simulink model "demo_simiplified_2"  (R2022b)
settings: Solver=VariableStepAuto  StartTime=0.0  StopTime=sim_time  RelTol=1e-4  AbsTol=1e-4
model workspace (MATLAB code in the model file):
  | official_parameters_2
undefined symbols (not defined in the file or in its folder): cd1, cd2_1, cd2_2, gas_pipe_D, initial_system_T, mass_flow_cp, Max_tank_V, N2_T, sim_time, stack_area, stack_mea_rho, stack_num_cells, stack_num_channels, stack_t_gdl_A, stack_t_gdl_C, stack_t_membrane, stack_w_channels, tank_plant_area, water_pipe_D
libraries: fl_lib x25, nesl_utility x4, SimscapeFluids_lib x1
CloseFcn:
  | try,close(h1_ssc_electrolyzer),end
  | clear h1_ssc_electrolyzer
  | try,close(h2_ssc_electrolyzer),end
  | clear h2_ssc_electrolyzer
  | try,close(h3_ssc_electrolyzer),end
  | clear h3_ssc_electrolyzer
  | 
  | clear tout simlog_ssc_electrolyzer
Description:
  | PEM Electrolysis System
settings Model: Creator=The MathWorks, Inc.  LastModifiedBy=15713
settings SolverCC: AutoScaleAbsTol=off  MaxConsecutiveMinStep=8  AlgebraicLoopSolver=TrustRegion  MaxZcPerStep=1
settings DataIOCC: ReturnWorkspaceOutputs=off
settings DebuggingCC: UnconnectedInputMsg=warning  UnconnectedOutputMsg=warning  UnconnectedLineMsg=warning  SymbolicDimsDataTypeCodeGenerationDiagnostic=none  SFMachineParentedDataDiag=warning
settings ModelReferenceCC: EnableRefExpFcnMdlSchedulingChecks=on
settings SFSimCC: CustomCodeUndefinedFunction=UseInterfaceOnly
settings RTWCC: DLArmComputeVersion=19.05
settings SimscapeCC: SimscapeLogType=all  SimscapeLogSimulationStatistics=on  SimscapeLogName=simlog_ssc_electrolyzer  SimscapeLogDataHistory=10000

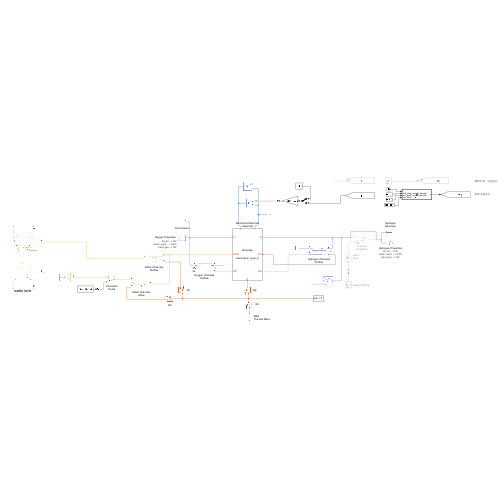
[thumbnail: Simulink's stored preview of the top-level diagram]
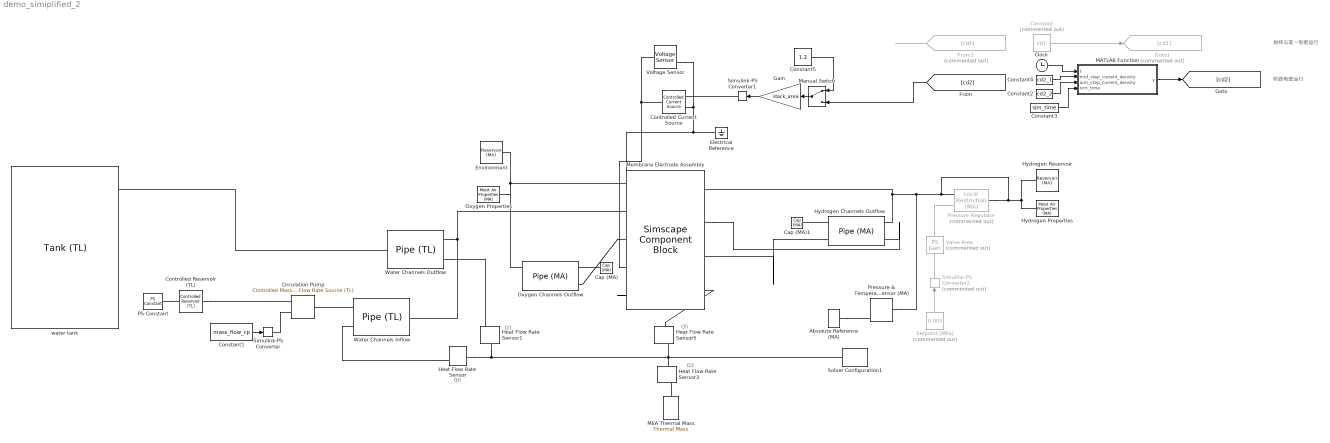
== system demo_simiplified_2 ==
  note: 始终以某一电密运行
  note: Q1
  note: Q0
  note: Q3
  note: Q5
  note: 阶跃电密运行
  Absolute Reference (MA) : fl_lib/Moist Air/Elements/Absolute Reference (MA)
  Cap (MA) : fl_lib/Moist Air/Elements/Cap (MA)  p_specify=off  p_priority=None  p=0.1 MPa  p_nominal_specify=off  p_nominal_unit=MPa  p_nominal_value=1  T_specify=off  T_priority=None  T=300 K  T_nominal_specify=off  T_nominal_unit=K  T_nominal_value=1  x_w_specify=off  x_w_priority=None  x_w=0  x_w_nominal_specify=off  x_w_nominal_unit=1  x_w_nominal_value=1  x_g_specify=off  x_g_priority=None  x_g=0  x_g_nominal_specify=off  x_g_nominal_unit=1  x_g_nominal_value=1
      settings: InternalSimscapePortConfiguration="{\"Bottom\":[],\"Left\":[{\"id\":\"A\",\"label\":\"\",\"type\":\"foundation.moist_air.moist_air\"}],\"Right\":[],\"Top\":[]}"
  Cap (MA)1 : fl_lib/Moist Air/Elements/Cap (MA)  p_specify=off  p_priority=None  p=0.1 MPa  p_nominal_specify=off  p_nominal_unit=MPa  p_nominal_value=1  T_specify=on  T_priority=High  T=initial_system_T degC  T_nominal_specify=off  T_nominal_unit=K  T_nominal_value=1  x_w_specify=off  x_w_priority=None  x_w=0  x_w_nominal_specify=off  x_w_nominal_unit=1  x_w_nominal_value=1  x_g_specify=off  x_g_priority=None  x_g=0  x_g_nominal_specify=off  x_g_nominal_unit=1  x_g_nominal_value=1
      settings: InternalSimscapePortConfiguration="{\"Bottom\":[],\"Left\":[{\"id\":\"A\",\"label\":\"\",\"type\":\"foundation.moist_air.moist_air\"}],\"Right\":[],\"Top\":[]}"
  Circulation Pump : fl_lib/Thermal Liquid/Sources/Controlled Mass Flow Rate Source (TL)  area=pi*water_pipe_D^2/4 m^2
      settings: InternalSimscapePortConfiguration="{\"Bottom\":[],\"Left\":[{\"id\":\"A\",\"label\":\"A\",\"type\":\"foundation.thermal_liquid.thermal_liquid\"},{\"id\":\"M\",\"label\":\"M\",\"type\":\"input\"}],\"Right\":[{\"id\":\"B\",\"label\":\"B\",\"type\":\"foundation.thermal_liquid.thermal_liquid\"}],\"Top\":[]}"
  Clock : Clock
  Constant : Constant  Commented=on  Value=cd1
  Constant1 : Constant  Value=mass_flow_cp
  Constant2 : Constant  Value=cd2_2
  Constant3 : Constant  Value=sim_time
  Constant4 : Constant  Value=cd2_1
  Constant5 : Constant  Value=1.2
  Controlled Current Source : fl_lib/Electrical/Electrical Sources/Controlled Current Source
  Controlled Reservoir (TL) : fl_lib/Thermal Liquid/Elements/Controlled Reservoir (TL)  pressure_spec=foundation.enum.pressure_spec.atmospheric  reservoir_pressure=0.101325 MPa  area=pi*water_pipe_D^2/4 m^2
      settings: InternalSimscapePortConfiguration="{\"Bottom\":[],\"Left\":[{\"id\":\"A\",\"label\":\"A\",\"type\":\"foundation.thermal_liquid.thermal_liquid\"}],\"Right\":[{\"id\":\"T_in\",\"label\":\"T\",\"type\":\"input\"}],\"Top\":[]}"
  Electrical Reference : fl_lib/Electrical/Electrical Elements/Electrical Reference
  Environment : fl_lib/Moist Air/Elements/Reservoir (MA)  pressure_spec=foundation.enum.pressure_spec.specified  reservoir_pressure=env_p MPa  temperature_spec=foundation.enum.temperature_spec.specified  reservoir_temperature=initial_system_T degC  moisture_spec=foundation.enum.moisture_spec.mole_fraction  reservoir_RH=0.5  reservoir_x_w=0.01  reservoir_y_w=0  reservoir_HR=0.01  trace_gas_spec=foundation.enum.trace_gas_spec.mole_fraction  reservoir_x_g=0.001  reservoir_y_g=1  RH_ws=1  area_A=pi*gas_pipe_D^2/4 m^2
  From1 : From  Commented=on  GotoTag=cd1
  Gain : Gain  Gain=stack_area
  Goto1 : Goto  Commented=on  GotoTag=cd1
  Heat Flow Rate Sensor{,1,3,5} (4 alike) : fl_lib/Thermal/Thermal Sensors/Heat Flow Rate Sensor
  Hydrogen Reservoir : fl_lib/Moist Air/Elements/Reservoir (MA)  pressure_spec=foundation.enum.pressure_spec.specified  reservoir_pressure=env_p MPa  temperature_spec=foundation.enum.temperature_spec.specified  reservoir_temperature=20 degC  moisture_spec=foundation.enum.moisture_spec.mole_fraction  reservoir_RH=0.5  reservoir_x_w=0.01  reservoir_y_w=0  reservoir_HR=0.01  trace_gas_spec=foundation.enum.trace_gas_spec.mole_fraction  reservoir_x_g=0.001  reservoir_y_g=1  RH_ws=1  area_A=pi*gas_pipe_D^2/4 m^2
  Hydrogen Channels Outflow : fl_lib/Moist Air/Elements/Pipe (MA)  length=sqrt(stack_area) cm  area=stack_w_channels^2 * stack_num_channels * stack_num_cells cm^2  Dh=stack_w_channels cm  length_add=1 cm  roughness=15e-6 m  Re_lam=2000  Re_tur=4000  shape_factor=64  Nu_lam=3.66  wall_condensation=simscape.enum.onoff.off  RH_ws=1  time_constant=1e-3 s  moisture_trace_gas_source=foundation.enum.moisture_trace_gas_source.controlled  moisture_source_spec=foundation.enum.moisture_source_spec.vapor  moisture_mass_flow=0 kg/s  moisture_temperature_spec=foundation.enum.temperature_spec.atmospheric  moisture_temperature=293.15 K  trace_gas_mass_flow=0 kg/s  trace_gas_temperature_spec=foundation.enum.temperature_spec.atmospheric  trace_gas_temperature=293.15 K  p_I_specify=on  p_I_priority=High  p_I=env_p MPa  p_I_nominal_specify=off  p_I_nominal_unit=MPa  p_I_nominal_value=1  T_I_specify=on  T_I_priority=High  T_I=initial_system_T degC  T_I_nominal_specify=off  T_I_nominal_unit=K  T_I_nominal_value=1  RH_I_specify=on  RH_I_priority=None  RH_I=0  RH_I_nominal_specify=off  RH_I_nominal_unit=1  RH_I_nominal_value=1  x_w_I_specify=off  x_w_I_priority=None  x_w_I=0  x_w_I_nominal_specify=off  x_w_I_nominal_unit=1  x_w_I_nominal_value=1  y_w_I_specify=on  y_w_I_priority=High  y_w_I=0  y_w_I_nominal_specify=off  y_w_I_nominal_unit=1  y_w_I_nominal_value=1  HR_I_specify=off  HR_I_priority=None  HR_I=0  HR_I_nominal_specify=off  HR_I_nominal_unit=1  HR_I_nominal_value=1  x_g_I_specify=on  x_g_I_priority=None  x_g_I=1  x_g_I_nominal_specify=off  x_g_I_nominal_unit=1  x_g_I_nominal_value=1  y_g_I_specify=on  y_g_I_priority=High  y_g_I=1  y_g_I_nominal_specify=off  y_g_I_nominal_unit=1  y_g_I_nominal_value=1
      settings: InternalSimscapePortConfiguration="{\"Bottom\":[],\"Left\":[{\"id\":\"A\",\"label\":\"A\",\"type\":\"foundation.moist_air.moist_air\"},{\"id\":\"H\",\"label\":\"H\",\"type\":\"foundation.thermal.thermal\"},{\"id\":\"S\",\"label\":\"S\",\"type\":\"foundation.moist_air.moist_air_source\"}],\"Right\":[{\"id\":\"B\",\"label\":\"B\",\"type\":\"foundation.moist_air.moist_air\"},{\"id\":\"W\",\"label\":\"W\",\"type\":\"output\"},{\"id\":\"F\",\"label\":\"F\",\"type\":\"output\"}],\"Top\":[]}"
  Hydrogen Properties : fl_lib/Moist Air/Utilities/Moist Air Properties (MA)  R_a=N2_R J/kg/K  T_TLU=N2_T degC  h_a_TLU=N2_h kJ/kg  mu_a_TLU=N2_mu s*uPa  k_a_TLU=N2_k mW/m/K  p_min=1 kPa  p_max=inf MPa  T_min=min(N2_T) degC  T_max=max(N2_T) degC  p_atm=0.101325 MPa  T_atm=20 degC  R_w=461.523 J/kg/K  p_ws_TLU=[1.71168953425982e-06; 3.93770601979424e-06; 1.28411717710344e-05; 3.80051394873809e-05; .00010323902900209; .000259873810798063; .000401741022116384; .000437454836117844; .000476040820618202; .000517704666185737; .000562664883741207; .000611212677444345; .000657088049117899; .000705987905898279; .000758082381149132; .000813549384183233; .000872574861129522; .00122818386934022; .0023392147667769; .00424668834054807; .00738442748706953; .0123512704340234; .0199458019246787; .0312006356960619; .0474147199263783; .0701823607447713; .10141797792131; .143375967241115; .198665399739302; .270259606559999; .361500961984849; .476101381081492; .618139196722055; .792053183687694; 1.0026345688121; 1.25501792086105; 1.55467186826983; 1.90739066433297; 2.31928772772542; 2.79679245576864; 3.34665187151016; 3.97593907083533; 4.69207105435535; 5.5028394740883; 6.41645928168037; 7.4416425436169; 8.58770832955728; 9.86474556030261; 11.2838558865497; 12.8575218898034; 14.6001810568052; 16.5291642526045] MPa  h_w_vap_TLU=[2836.88241275372; 2837.81392500514; 2838.63937175807; 2838.7309929628; 2838.06905313927; 2836.62597341095; 2835.60023952573; 2835.37006381376; 2835.13143158077; 2834.88429145066; 2834.62859062897; 2500.93420564316; 2498.55329907119; 2496.17495082036; 2493.79885912205; 2491.42474723191; 2489.05236104642; 2477.20875029194; 2453.54955988604; 2429.83856603313; 2406.00136954922; 2381.97406342174; 2357.69101156389; 2333.08088387814; 2308.06565480412; 2282.56034405021; 2256.47287422313; 2229.70428017508; 2202.14968030993; 2173.69998896199; 2144.24368406447; 2113.66758247452; 2081.85585110571; 2048.68725710494; 2014.03141249899; 1977.7449923284; 1939.66849592886; 1899.62342931686; 1857.40930169838; 1812.79975416601; 1765.53721731251; 1715.32525772152; 1661.81700477787; 1604.59703745016; 1543.1534616334; 1476.83692476464; 1404.80240352424; 1325.92091736114; 1238.61667822208; 1140.5102987018; 1027.62017777647; 892.733785613825] kJ/kg  h_w_TLU=[2396.55944251649; 2408.68643343608; 2427.1988031141; 2445.702165897; 2464.18429108356; 2482.62529466839; 2491.82135326629; 2493.6580151792; 2495.49372578218; 2497.32843835745; 2499.16210446923; 2500.99462758899; 2502.83092214066; 2504.6665223621; 2506.50140563013; 2508.335548891; 2510.16892865793; 2519.32352241995; 2537.56068088674; 2555.67742615292; 2573.6403223998; 2591.4109179101; 2608.9455037701; 2626.19492016262; 2643.10444358428; 2659.61377634497; 2675.58278696023; 2696.1846256545; 2716.49989553741; 2736.6235210957; 2756.61216047011; 2776.50561773853; 2796.33378922508; 2816.11979583049; 2835.88181423877; 2855.63430574511; 2875.38889327595; 2895.15500577172; 2914.94035964689; 2934.75132290228; 2954.59319330244; 2974.47041285505; 2994.38673458964; 3014.34535328009; 3034.34900867103; 3054.40006755764; 3074.50058946898; 3094.65237953784; 3114.85703128106; 3135.11596137801; 3155.43043805905; 3175.80160435813] kJ/kg  mu_w_TLU=[6.81365662228272; 7.04953750742707; 7.40970098298307; 7.76991278093907; 8.13017290129507; 8.49048134405107; 8.67065368632907; 8.70668960445667; 8.74272600580827; 8.77876289038387; 8.81480025818347; 8.85083810920707; 8.88687644345467; 8.92291526092627; 8.95895456162187; 8.99499434554147; 9.03103461268507; 9.21124319676307; 9.57169660671907; 9.93219833907507; 10.2927483938311; 10.6533467709871; 11.0139934705431; 11.3746884924991; 11.7354318368551; 12.0962235036111; 12.4570634927671; 12.8179518043231; 13.1788884382791; 13.5398733946351; 13.9009066733911; 14.2619882745471; 14.6231181981031; 14.9842964440591; 15.3455230124151; 15.7067979031711; 16.0681211163271; 16.4294926518831; 16.7909125098391; 17.1523806901951; 17.5138971929511; 17.8754620181071; 18.2370751656631; 18.5987366356191; 18.9604464279751; 19.3222045427311; 19.6840109798871; 20.0458657394431; 20.4077688213991; 20.7697202257551; 21.1317199525111; 21.4937680016671] s*uPa  k_w_TLU=[11.46288215976; 11.941997488935; 12.676358586935; 13.414208884935; 14.155548382935; 14.900377080935; 15.274099879935; 15.348949115735; 15.423833243535; 15.498752263335; 15.573706175135; 15.648694978935; 15.723718674735; 15.798777262535; 15.873870742335; 15.948999114135; 16.024162377935; 16.400502076935; 17.155798374935; 17.914583872935; 18.676858570935; 19.442622468935; 20.211875566935; 20.984617864935; 21.760849362935; 22.540570060935; 23.323779958935; 24.110479056935; 24.900667354935; 25.694344852935; 26.491511550935; 27.292167448935; 28.096312546935; 28.903946844935; 29.715070342935; 30.529683040935; 31.347784938935; 32.169376036935; 32.994456334935; 33.823025832935; 34.655084530935; 35.490632428935; 36.329669526935; 37.172195824935; 38.018211322935; 38.867716020935; 39.720709918935; 40.577193016935; 41.437165314935; 42.300626812935; 43.167577510935; 44.038017408935] mW/m/K  D_w=25 mm^2/s  trace_gas_model=foundation.enum.trace_gas_model.track_properties  R_g=H2_R J/kg/K  h_g_TLU=H2_h kJ/kg  mu_g_TLU=H2_mu s*uPa  k_g_TLU=H2_k mW/m/K  D_g=H2_D mm^2/s
      settings: AttributesFormatString=|
      | dry air --> N2
      | water vapor --> H2O
      | trace gas --> H2
  MATLAB Function : MATLAB Function  TreatAsAtomicUnit=on
  MEA Thermal Mass : fl_lib/Thermal/Thermal Elements/Thermal Mass  mass=stack_mea_rho * stack_area*1e-4 * (stack_t_membrane + stack_t_gdl_A + stack_t_gdl_C)*1e-6 * stack_num_cells kg  sp_heat=stack_mea_cp J/kg/K  num_ports=foundation.enum.numPorts2.one  T_specify=on  T_priority=High  T=initial_system_T degC  T_nominal_specify=off  T_nominal_unit=K  T_nominal_value=1  Q_specify=off  Q_priority=None  Q=0 W  Q_nominal_specify=off  Q_nominal_unit=W  Q_nominal_value=1
  Manual Switch : ManualSwitch
  Membrane Electrode Assembly : SimscapeComponentBlock  SourceFile=electrolyzer_work_2  ComponentPath=electrolyzer_work_2  ComponentVariants="[\"electrolyzer_work_2\"]"  ComponentVariantNames="[\"electrolyzer_work_2\"]"  ClassName=electrolyzer_work_2  SchemaVersion=1  N_cell=50  area_cell=280 cm^2  t_membrane=125 um  ioref=8e-05 A/cm^2  alpha=0.5  ohm_effi=1  ilim=10 A/cm^2  t_gdl_A=25 um  t_gdl_C=250 um  D_H2O_gdl_A=0.07 cm^2/s  D_H2O_gdl_C=0.07 cm^2/s  rho_membrane=2000 kg/m^3  M_membrane=1.1 kg/mol  D0=4.9 cm^2/s  Ed=16510 J/mol  H2_solubility_in_H2O_T=[273.15 : 10 : 373.15] K  H2_solubility_in_H2O_P=[1, 25, 50, 75, 100, 150, 200, 300, 400, 500, 600, 700, 800, 900, 1000]' bar  H2_solubility_in_H2O=[9.45e-12, 8.58e-12, 7.92e-12, 7.51e-12, 7.28e-12, 7.16e-12, 7.14e-12, 7.21e-12, 7.4e-12, 7.72e-12, 8.13e-12; 9.45e-12, 8.58e-12, 7.92e-12, 7.51e-12, 7.28e-12, 7.16e-12, 7.14e-12, 7.21e-12, 7.4e-12, 7.72e-12, 8.13e-12; 9.41e-12, 8.53e-12, 7.88e-12, 7.46e-12, 7.23e-12, 7.12e-12, 7.13e-12, 7.2e-12, 7.38e-12, 7.68e-12, 8.03e-12; 9.4e-12, 8.53e-12, 7.87e-12, 7.46e-12, 7.23e-12, 7.12e-12, 7.11e-12, 7.29e-12, 7.36e-12, 7.62e-12, 7.96e-12; 9.38e-12, 8.51e-12, 7.86e-12, 7.44e-12, 7.21e-12, 7.1e-12, 7.09e-12, 7.17e-12, 7.35e-12, 7.6e-12, 7.95e-12; 9.3e-12, 8.43e-12, 7.78e-12, 7.36e-12, 7.14e-12, 7.03e-12, 7.02e-12, 7.11e-12, 7.29e-12, 7.56e-12, 7.87e-12; 9.22e-12, 8.36e-12, 7.7e-12, 7.29e-12, 7.07e-12, 6.97e-12, 6.98e-12, 7.06e-12, 7.23e-12, 7.49e-12, 7.8e-12; 9.01e-12, 8.19e-12, 7.57e-12, 7.19e-12, 6.97e-12, 6.89e-12, 6.89e-12, 6.97e-12, 7.14e-12, 7.4e-12, 7.66e-12; 8.82e-12, 8.04e-12, 7.45e-12, 7.08e-12, 6.87e-12, 6.79e-12, 6.8e-12, 6.88e-12, 7.04e-12, 7.27e-12, 7.53e-12; 8.66e-12, 7.91e-12, 7.33e-12, 6.98e-12, 6.79e-12, 6.7e-12, 6.72e-12, 6.8e-12, 6.94e-12, 7.16e-12, 7.42e-12; 8.53e-12, 7.79e-12, 7.23e-12, 6.89e-12, 6.7e-12, 6.62e-12, 6.62e-12, 6.7e-12, 6.84e-12, 7.09e-12, 7.33e-12; 8.41e-12, 7.7e-12, 7.15e-12, 6.81e-12, 6.62e-12, 6.54e-12, 6.55e-12, 6.62e-12, 6.77e-12, 6.98e-12, 7.24e-12; 8.26e-12, 7.57e-12, 7.05e-12, 6.73e-12, 6.54e-12, 6.46e-12, 6.47e-12, 6.55e-12, 6.7e-12, 6.91e-12, 7.14e-12; 8.1e-12, 7.44e-12, 6.96e-12, 6.65e-12, 6.47e-12, 6.4e-12, 6.4e-12, 6.47e-12, 6.62e-12, 6.82e-12, 7.04e-12; 7.93e-12, 7.32e-12, 6.87e-12, 6.57e-12, 6.42e-12, 6.34e-12, 6.34e-12, 6.41e-12, 6.55e-12, 6.74e-12, 6.95e-12] mol/(Pa*cm^3)  i_specify=off  i_priority=None  i=0 A  i_nominal_specify=off  i_nominal_unit=A  i_nominal_value=1  RH_acl_specify=off  RH_acl_priority=None  RH_acl=0.5  RH_acl_nominal_specify=off  RH_acl_nominal_unit=1  RH_acl_nominal_value=1  RH_ccl_specify=off  RH_ccl_priority=None  RH_ccl=0.5  RH_ccl_nominal_specify=off  RH_ccl_nominal_unit=1  RH_ccl_nominal_value=1  Q_specify=off  Q_priority=None  Q=0 kW  Q_nominal_specify=off  Q_nominal_unit=kW  Q_nominal_value=1  mdot_H2O_specify=off  mdot_H2O_priority=None  mdot_H2O=0 kg/s  mdot_H2O_nominal_specify=off  mdot_H2O_nominal_unit=kg/s  mdot_H2O_nominal_value=1  Phi_H2O_specify=off  Phi_H2O_priority=None  Phi_H2O=0 kW  Phi_H2O_nominal_specify=off  Phi_H2O_nominal_unit=kW  Phi_H2O_nominal_value=1
      settings: CopyFcn=simscape.engine.sli.internal.componentblockcallback(gcbh,'COPY')  PreCopyFcn=simscape.engine.sli.internal.componentblockcallback(gcbh,'PRECOPY')  PreDeleteFcn=simscape.engine.sli.internal.componentblockcallback(gcbh,'PREDELETE')  InternalSimscapePortConfiguration="{\"Bottom\":[{\"id\":\"H\",\"label\":\"H\",\"type\":\"foundation.thermal.thermal\"}],\"Left\":[{\"id\":\"A\",\"label\":\"A\",\"type\":\"foundation.moist_air.moist_air\"},{\"id\":\"H2O\",\"label\":\"H2O\",\"type\":\"foundation.thermal_liquid.thermal_liquid\"},{\"id\":\"O2\",\"label\":\"O2\",\"type\":\"foundation.moist_air.moist_air_source\"}],\"Right\":[{\"id\":\"C\",\"label\":\"C\",\"type\":\"foundation.moist_air.moist_air\"},{\"id\":\"FC\",\"label\":\"FC\",\"type\":\"input\"},{\"id\":\"H2\",\"label\":\"H2\",\"type\":\"foundation.moist_air.moist_air_source\"}],\"Top\":[{\"id\":\"An\",\"label\":\"+\",\"type\":\"foundation.electrical.electrical\"},{\"id\":\"Ca\",\"label\":\"-\",\"type\":\"foundation.electrical.electrical\"}]}"
      mask Type: This is customed electrolyzer
  Oxygen Channels Outflow : fl_lib/Moist Air/Elements/Pipe (MA)  length=sqrt(stack_area) cm  area=stack_w_channels^2 * stack_num_channels * stack_num_cells cm^2  Dh=stack_w_channels cm  length_add=1 m  roughness=15e-6 m  Re_lam=2000  Re_tur=4000  shape_factor=64  Nu_lam=3.66  wall_condensation=simscape.enum.onoff.off  RH_ws=1  time_constant=1e-3 s  moisture_trace_gas_source=foundation.enum.moisture_trace_gas_source.controlled  moisture_source_spec=foundation.enum.moisture_source_spec.vapor  moisture_mass_flow=0 kg/s  moisture_temperature_spec=foundation.enum.temperature_spec.atmospheric  moisture_temperature=293.15 K  trace_gas_mass_flow=0 kg/s  trace_gas_temperature_spec=foundation.enum.temperature_spec.atmospheric  trace_gas_temperature=293.15 K  p_I_specify=on  p_I_priority=High  p_I=env_p MPa  p_I_nominal_specify=off  p_I_nominal_unit=MPa  p_I_nominal_value=1  T_I_specify=on  T_I_priority=High  T_I=initial_system_T degC  T_I_nominal_specify=off  T_I_nominal_unit=K  T_I_nominal_value=1  RH_I_specify=on  RH_I_priority=None  RH_I=0  RH_I_nominal_specify=off  RH_I_nominal_unit=1  RH_I_nominal_value=1  x_w_I_specify=off  x_w_I_priority=None  x_w_I=0  x_w_I_nominal_specify=off  x_w_I_nominal_unit=1  x_w_I_nominal_value=1  y_w_I_specify=on  y_w_I_priority=High  y_w_I=0  y_w_I_nominal_specify=off  y_w_I_nominal_unit=1  y_w_I_nominal_value=1  HR_I_specify=off  HR_I_priority=None  HR_I=0  HR_I_nominal_specify=off  HR_I_nominal_unit=1  HR_I_nominal_value=1  x_g_I_specify=on  x_g_I_priority=None  x_g_I=1  x_g_I_nominal_specify=off  x_g_I_nominal_unit=1  x_g_I_nominal_value=1  y_g_I_specify=on  y_g_I_priority=High  y_g_I=1  y_g_I_nominal_specify=off  y_g_I_nominal_unit=1  y_g_I_nominal_value=1
      settings: InternalSimscapePortConfiguration="{\"Bottom\":[],\"Left\":[{\"id\":\"A\",\"label\":\"A\",\"type\":\"foundation.moist_air.moist_air\"},{\"id\":\"H\",\"label\":\"H\",\"type\":\"foundation.thermal.thermal\"},{\"id\":\"S\",\"label\":\"S\",\"type\":\"foundation.moist_air.moist_air_source\"}],\"Right\":[{\"id\":\"B\",\"label\":\"B\",\"type\":\"foundation.moist_air.moist_air\"},{\"id\":\"W\",\"label\":\"W\",\"type\":\"output\"},{\"id\":\"F\",\"label\":\"F\",\"type\":\"output\"}],\"Top\":[]}"
  Oxygen Properties : fl_lib/Moist Air/Utilities/Moist Air Properties (MA)  R_a=N2_R J/kg/K  T_TLU=N2_T degC  h_a_TLU=N2_h kJ/kg  mu_a_TLU=N2_mu s*uPa  k_a_TLU=N2_k mW/m/K  p_min=1 kPa  p_max=inf MPa  T_min=min(N2_T) degC  T_max=max(N2_T) degC  p_atm=0.101325 MPa  T_atm=20 degC  R_w=461.523 J/kg/K  p_ws_TLU=[1.71168953425982e-06; 3.93770601979424e-06; 1.28411717710344e-05; 3.80051394873809e-05; .00010323902900209; .000259873810798063; .000401741022116384; .000437454836117844; .000476040820618202; .000517704666185737; .000562664883741207; .000611212677444345; .000657088049117899; .000705987905898279; .000758082381149132; .000813549384183233; .000872574861129522; .00122818386934022; .0023392147667769; .00424668834054807; .00738442748706953; .0123512704340234; .0199458019246787; .0312006356960619; .0474147199263783; .0701823607447713; .10141797792131; .143375967241115; .198665399739302; .270259606559999; .361500961984849; .476101381081492; .618139196722055; .792053183687694; 1.0026345688121; 1.25501792086105; 1.55467186826983; 1.90739066433297; 2.31928772772542; 2.79679245576864; 3.34665187151016; 3.97593907083533; 4.69207105435535; 5.5028394740883; 6.41645928168037; 7.4416425436169; 8.58770832955728; 9.86474556030261; 11.2838558865497; 12.8575218898034; 14.6001810568052; 16.5291642526045] MPa  h_w_vap_TLU=[2836.88241275372; 2837.81392500514; 2838.63937175807; 2838.7309929628; 2838.06905313927; 2836.62597341095; 2835.60023952573; 2835.37006381376; 2835.13143158077; 2834.88429145066; 2834.62859062897; 2500.93420564316; 2498.55329907119; 2496.17495082036; 2493.79885912205; 2491.42474723191; 2489.05236104642; 2477.20875029194; 2453.54955988604; 2429.83856603313; 2406.00136954922; 2381.97406342174; 2357.69101156389; 2333.08088387814; 2308.06565480412; 2282.56034405021; 2256.47287422313; 2229.70428017508; 2202.14968030993; 2173.69998896199; 2144.24368406447; 2113.66758247452; 2081.85585110571; 2048.68725710494; 2014.03141249899; 1977.7449923284; 1939.66849592886; 1899.62342931686; 1857.40930169838; 1812.79975416601; 1765.53721731251; 1715.32525772152; 1661.81700477787; 1604.59703745016; 1543.1534616334; 1476.83692476464; 1404.80240352424; 1325.92091736114; 1238.61667822208; 1140.5102987018; 1027.62017777647; 892.733785613825] kJ/kg  h_w_TLU=[2396.55944251649; 2408.68643343608; 2427.1988031141; 2445.702165897; 2464.18429108356; 2482.62529466839; 2491.82135326629; 2493.6580151792; 2495.49372578218; 2497.32843835745; 2499.16210446923; 2500.99462758899; 2502.83092214066; 2504.6665223621; 2506.50140563013; 2508.335548891; 2510.16892865793; 2519.32352241995; 2537.56068088674; 2555.67742615292; 2573.6403223998; 2591.4109179101; 2608.9455037701; 2626.19492016262; 2643.10444358428; 2659.61377634497; 2675.58278696023; 2696.1846256545; 2716.49989553741; 2736.6235210957; 2756.61216047011; 2776.50561773853; 2796.33378922508; 2816.11979583049; 2835.88181423877; 2855.63430574511; 2875.38889327595; 2895.15500577172; 2914.94035964689; 2934.75132290228; 2954.59319330244; 2974.47041285505; 2994.38673458964; 3014.34535328009; 3034.34900867103; 3054.40006755764; 3074.50058946898; 3094.65237953784; 3114.85703128106; 3135.11596137801; 3155.43043805905; 3175.80160435813] kJ/kg  mu_w_TLU=[6.81365662228272; 7.04953750742707; 7.40970098298307; 7.76991278093907; 8.13017290129507; 8.49048134405107; 8.67065368632907; 8.70668960445667; 8.74272600580827; 8.77876289038387; 8.81480025818347; 8.85083810920707; 8.88687644345467; 8.92291526092627; 8.95895456162187; 8.99499434554147; 9.03103461268507; 9.21124319676307; 9.57169660671907; 9.93219833907507; 10.2927483938311; 10.6533467709871; 11.0139934705431; 11.3746884924991; 11.7354318368551; 12.0962235036111; 12.4570634927671; 12.8179518043231; 13.1788884382791; 13.5398733946351; 13.9009066733911; 14.2619882745471; 14.6231181981031; 14.9842964440591; 15.3455230124151; 15.7067979031711; 16.0681211163271; 16.4294926518831; 16.7909125098391; 17.1523806901951; 17.5138971929511; 17.8754620181071; 18.2370751656631; 18.5987366356191; 18.9604464279751; 19.3222045427311; 19.6840109798871; 20.0458657394431; 20.4077688213991; 20.7697202257551; 21.1317199525111; 21.4937680016671] s*uPa  k_w_TLU=[11.46288215976; 11.941997488935; 12.676358586935; 13.414208884935; 14.155548382935; 14.900377080935; 15.274099879935; 15.348949115735; 15.423833243535; 15.498752263335; 15.573706175135; 15.648694978935; 15.723718674735; 15.798777262535; 15.873870742335; 15.948999114135; 16.024162377935; 16.400502076935; 17.155798374935; 17.914583872935; 18.676858570935; 19.442622468935; 20.211875566935; 20.984617864935; 21.760849362935; 22.540570060935; 23.323779958935; 24.110479056935; 24.900667354935; 25.694344852935; 26.491511550935; 27.292167448935; 28.096312546935; 28.903946844935; 29.715070342935; 30.529683040935; 31.347784938935; 32.169376036935; 32.994456334935; 33.823025832935; 34.655084530935; 35.490632428935; 36.329669526935; 37.172195824935; 38.018211322935; 38.867716020935; 39.720709918935; 40.577193016935; 41.437165314935; 42.300626812935; 43.167577510935; 44.038017408935] mW/m/K  D_w=25 mm^2/s  trace_gas_model=foundation.enum.trace_gas_model.track_properties  R_g=O2_R J/kg/K  h_g_TLU=O2_h kJ/kg  mu_g_TLU=O2_mu s*uPa  k_g_TLU=O2_k mW/m/K  D_g=O2_D mm^2/s
      settings: AttributesFormatString=|
      | dry air --> N2
      | water vapor --> H2O
      | trace gas --> O2
  PS Constant : fl_lib/Physical Signals/Sources/PS Constant  constant=323.15 K
  Pressure Regulator : fl_lib/Moist Air/Elements/Local Restriction (MA)  Commented=on  restriction_type=foundation.enum.restriction_type.variable  restriction_area=0.001 m^2  min_area=pi*(1e-4*gas_pipe_D)^2/4 m^2  max_area=pi*(0.9*gas_pipe_D)^2/4 m^2  area=pi*gas_pipe_D^2/4 m^2  Cd=0.64  B_lam=0.999
  Pressure & Temperature Sensor (MA) : fl_lib/Moist Air/Sensors/Pressure & Temperature Sensor (MA)
      settings: InternalSimscapePortConfiguration="{\"Bottom\":[],\"Left\":[{\"id\":\"A\",\"label\":\"A\",\"type\":\"foundation.moist_air.moist_air\"}],\"Right\":[{\"id\":\"B\",\"label\":\"B\",\"type\":\"foundation.moist_air.moist_air\"},{\"id\":\"P\",\"label\":\"P\",\"type\":\"output\"},{\"id\":\"T\",\"label\":\"T\",\"type\":\"output\"}],\"Top\":[]}"
  Setpoint [MPa] : Constant  Commented=on  Value=0.005
  Simulink-PS Converter : nesl_utility/Simulink-PS Converter  PhysicalDomain=network_engine_domain  SubClassName=ps_input  LeftPortType=input  RightPortType=output  PseudoPeriodic=off  Frequencies=[]  NoiseDistribution=none  NoiseParameters=[]  Unit=1  AffineConversion=off  FilteringAndDerivatives=provide  SimscapeFilterOrder=1  InputFilterTimeConstant=0.001  UdotUserProvided=0
  Simulink-PS Converter1 : nesl_utility/Simulink-PS Converter  PhysicalDomain=network_engine_domain  SubClassName=ps_input  LeftPortType=input  RightPortType=output  PseudoPeriodic=off  Frequencies=[]  NoiseDistribution=none  NoiseParameters=[]  Unit=1  AffineConversion=off  FilteringAndDerivatives=provide  SimscapeFilterOrder=1  InputFilterTimeConstant=0.001  UdotUserProvided=0
  Simulink-PS Converter2 : nesl_utility/Simulink-PS Converter  Commented=on  PhysicalDomain=network_engine_domain  SubClassName=ps_input  LeftPortType=input  RightPortType=output  PseudoPeriodic=off  Frequencies=[]  NoiseDistribution=none  NoiseParameters=[]  Unit=1  AffineConversion=off  FilteringAndDerivatives=provide  SimscapeFilterOrder=1  InputFilterTimeConstant=0.001  UdotUserProvided=0
  Solver Configuration1 : nesl_utility/Solver Configuration  PhysicalDomain=network_engine_domain  SubClassName=solver  LeftPortType=input  RightPortType=generic  Tones=[]  Harmonics=[]  SimulateNoise=off  Profile=off  UseLocalSampling=off  EnableSwitchedLinearOptims=on  FrequencyDomain=off  UseCCode=off  RelTol=0.001  AbsTol=0.001  MinStep=1e-09  ToWorkspace=off  RevertToSquareIcSolve=off  NumHomotopyIterations=100  PhasorMode=off  PhasorModeNumHarmonics=1  ConsistencySolver=NEWTON_XTOL_AFTER_FTOL  IndexReductionMethod=DerivativeReplacement  DoDC=off  ResidualTolerance=1e-09  ConsistencyTolSource=GLOBAL  ConsistencyAbsTol=0.001  ConsistencyRelTol=0.001  ConsistencyTolFactor=0.001  UseLocalSolver=off  LocalSolverChoice=NE_BACKWARD_EULER_ADVANCER  ResolveIndetEquations=on  FunctionEvalNumThread=1  LocalSolverSampleTime=0.001  DoFixedCost=off  MaxNonlinIter=3  MaxModeIter=2  ComputeImpulses=off  ImpulseIterations=2  LinearAlgebra=auto  LinearAlgebraNumThread=0  EquationFormulation=NE_TIME_EF  DelaysMemoryBudget=1024  AutomaticFiltering=on  FilteringTimeConstant=0.001  PartitionStorageMethod=AS_NEEDED  PartitionMemoryBudget=1024  PartitionMethod=ROBUST
  Valve Area : fl_lib/Physical Signals/Functions/PS Gain  Commented=on  gain=pi*(0.9*gas_pipe_D)^2/4 m^2
  Voltage Sensor : fl_lib/Electrical/Electrical Sensors/Voltage Sensor
  Water Channels Inflow : fl_lib/Thermal Liquid/Elements/Pipe (TL)  length=sqrt(stack_area) / 2 cm  area=stack_w_channels^2 * stack_num_channels * stack_num_cells cm^2  Dh=stack_w_channels cm  length_add=1 cm  roughness=15e-6 m  Re_lam=2000  Re_tur=4000  shape_factor=64  Nu_lam=3.66  dynamic_compressibility=simscape.enum.onoff.on  inertia=simscape.enum.onoff.off  p0=env_p MPa  T0=initial_system_T degC  mdot0=0 kg/s
  Water Channels Outflow : fl_lib/Thermal Liquid/Elements/Pipe (TL)  length=sqrt(stack_area) / 2 cm  area=stack_w_channels^2 * stack_num_channels * stack_num_cells cm^2  Dh=stack_w_channels cm  length_add=1 cm  roughness=15e-6 m  Re_lam=2000  Re_tur=4000  shape_factor=64  Nu_lam=3.66  dynamic_compressibility=simscape.enum.onoff.on  inertia=simscape.enum.onoff.off  p0=env_p MPa  T0=initial_system_T degC  mdot0=0 kg/s
  water tank : SimscapeFluids_lib/Thermal Liquid/Tanks & Accumulators/Tank (TL)  num_inlet=fluids.thermal_liquid.tanks_accumulators.enum.NumInlet.Two  pressure_spec=foundation.enum.pressure_spec.specified  tank_pressure=env_p MPa  volume_spec=fluids.thermal_liquid.tanks_accumulators.enum.TankVolumeSpec.Constant  tank_area=tank_plant_area m^2  level_TLU=[0, 3, 5] m  volume_TLU=[0, 4, 6] m^3  inlet_height_A=0.1 m  inlet_area_A=0.01 m^2  inlet_heights_AB=[Max_tank_V/tank_plant_area, 0] m  inlet_areas_AB=[pi*water_pipe_D^2/4,pi*water_pipe_D^2/4] m^2  inlet_heights_ABC=[Max_tank_V/tank_plant_area, Max_tank_V/tank_plant_area, 0] m  inlet_areas_ABC=(pi*water_pipe_D^2/4)*ones(1,3) m^2  inlet_heights_ABCD=0.1 * ones(1, 4) m  inlet_areas_ABCD=0.01 * ones(1, 4) m^2  inlet_heights_ABCDE=0.1 * ones(1, 5) m  inlet_areas_ABCDE=0.01 * ones(1, 5) m^2  inlet_heights_ABCDEF=0.1 * ones(1, 6) m  inlet_areas_ABCDEF=0.01 * ones(1, 6) m^2  level_check=simscape.enum.assert.action.none  capacity_check=simscape.enum.assert.action.warn  max_capacity=Max_tank_V m^3  g=9.81 m/s^2  level_specify=on  level_priority=High  level=Initial_L_level m  level_nominal_specify=off  level_nominal_unit=m  level_nominal_value=1  volume_specify=off  volume_priority=None  volume=1 m^3  volume_nominal_specify=off  volume_nominal_unit=m^3  volume_nominal_value=1  mass_specify=off  mass_priority=None  mass=5000 kg  mass_nominal_specify=off  mass_nominal_unit=kg  mass_nominal_value=1  T_I_specify=on  T_I_priority=High  T_I=initial_system_T degC  T_I_nominal_specify=off  T_I_nominal_unit=K  T_I_nominal_value=1
      settings: LogSimulationData=on  InternalSimscapePortConfiguration="{\"Bottom\":[{\"id\":\"H\",\"label\":\"H\",\"type\":\"foundation.thermal.thermal\"},{\"id\":\"T_out\",\"label\":\"T\",\"type\":\"output\"}],\"Left\":[{\"id\":\"A\",\"label\":\"A\",\"type\":\"foundation.thermal_liquid.thermal_liquid\"},{\"id\":\"B\",\"label\":\"B\",\"type\":\"foundation.thermal_liquid.thermal_liquid\"}],\"Right\":[],\"Top\":[{\"id\":\"V_out\",\"label\":\"V\",\"type\":\"output\"},{\"id\":\"L_out\",\"label\":\"L\",\"type\":\"output\"}]}"
  wires:
  Constant1/1 -> Simulink-PS Converter/1
  Manual Switch/1 -> Gain/1
  Gain/1 -> Simulink-PS Converter1/1
  Constant/1 -> Goto1/1
  Clock/1 -> MATLAB Function/1(t)
  MATLAB Function/1(y) -> [cd2]
  Constant2/1 -> MATLAB Function/3(aim_step_current_density)
  Constant4/1 -> MATLAB Function/2(mid_step_current_density)
  [cd2] -> Manual Switch/2
  Setpoint [MPa]/1 -> Simulink-PS Converter2/1
  Constant3/1 -> MATLAB Function/4(sim_time)
  From1/1 -> ?
  Constant5/1 -> Manual Switch/1
  connections:
  Simulink-PS Converter/RConn1 -- Circulation Pump/LConn2
  Membrane Electrode Assembly/LConn1 -- Oxygen Channels Outflow/RConn1 -- Oxygen Properties/RConn1 -- Environment/LConn1
  Water Channels Outflow/LConn1 -- Water Channels Inflow/RConn1 -- Membrane Electrode Assembly/LConn2
  Oxygen Channels Outflow/LConn1 -- Cap (MA)/LConn1
  Membrane Electrode Assembly/LConn3 -- Oxygen Channels Outflow/LConn3
  Solver Configuration1/RConn1 -- Heat Flow Rate Sensor/LConn1 -- Heat Flow Rate Sensor1/LConn1 -- Heat Flow Rate Sensor3/LConn1 -- Heat Flow Rate Sensor5/RConn2
  Voltage Sensor/LConn1 -- Controlled Current Source/LConn1 -- Membrane Electrode Assembly/LConn4
  Membrane Electrode Assembly/RConn2 -- Hydrogen Channels Outflow/RConn3
  Hydrogen Channels Outflow/LConn3 -- Membrane Electrode Assembly/RConn3
  Hydrogen Channels Outflow/LConn1 -- Cap (MA)1/LConn1
  Controlled Current Source/RConn2 -- Electrical Reference/LConn1 -- Membrane Electrode Assembly/LConn5 -- Voltage Sensor/RConn2
  Simulink-PS Converter1/RConn1 -- Controlled Current Source/RConn1
  Water Channels Inflow/LConn2 -- Heat Flow Rate Sensor/RConn2
  Water Channels Outflow/LConn2 -- Heat Flow Rate Sensor1/RConn2
  Membrane Electrode Assembly/RConn4 -- Heat Flow Rate Sensor5/LConn1
  MEA Thermal Mass/LConn1 -- Heat Flow Rate Sensor3/RConn2
  Water Channels Outflow/RConn1 -- water tank/LConn1
  Water Channels Inflow/LConn1 -- Circulation Pump/RConn1
  Controlled Reservoir (TL)/LConn1 -- Circulation Pump/LConn1
  PS Constant/RConn1 -- Controlled Reservoir (TL)/RConn1
  Valve Area/RConn1 -- Pressure Regulator/LConn2
  Simulink-PS Converter2/RConn1 -- Valve Area/LConn1
  Hydrogen Channels Outflow/RConn1 -- Pressure Regulator/LConn1 -- Hydrogen Reservoir/LConn1 -- Hydrogen Properties/RConn1 -- Pressure Regulator/RConn1 -- Pressure & Temperature Sensor (MA)/LConn1 -- Membrane Electrode Assembly/RConn1
  Absolute Reference (MA)/LConn1 -- Pressure & Temperature Sensor (MA)/RConn1

== matlab function demo_simiplified_2/MATLAB Function ==
  data: t input; mid_step_current_density input; y output; aim_step_current_density input; sim_time input
function y = fcn(t,mid_step_current_density ,aim_step_current_density,sim_time)
    if t<50
        y = 0;
    elseif 50<=t&&t<=((sim_time-50)/2+50)
        y = mid_step_current_density;
    else 
        y = aim_step_current_density;

    end
